simulink model "OPModel"  (R2014a)
settings: Solver=ode45  StartTime=0.0  StopTime=10  RelTol=1e-3
values from neighbouring files (symbols this model uses):
  K1 = A*x+B*r    [RongKutta.m]
  K2 = A*(x+h*K1/2)+B*r    [RongKutta.m]
undefined symbols (not defined in the file or in its folder): Kd, Ki, Kp
settings Model: Creator=李广文  LastModifiedBy=李广文

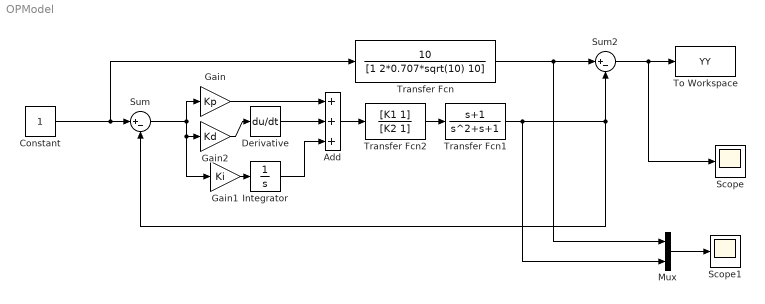
== system OPModel ==
  Add : Sum  Inputs=+++
  Constant : Constant
  Derivative : Derivative
  Gain : Gain  Gain=Kp
  Gain1 : Gain  Gain=Ki
  Gain2 : Gain  Gain=Kd
  Integrator : Integrator
  Mux : Mux  Inputs=2
  Scope : Scope
  Scope1 : Scope
      settings: YMin=0  YMax=1.5
  Sum : Sum  Inputs=|+-
  Sum2 : Sum  Inputs=|+-
  To Workspace : ToWorkspace  VariableName=YY  SampleTime=-1
  Transfer Fcn : TransferFcn  Numerator=[10]  Denominator=[1 2*0.707*sqrt(10) 10]
  Transfer Fcn1 : TransferFcn  Numerator=[1 1]  Denominator=[1 1 1]
  Transfer Fcn2 : TransferFcn  Numerator=[K1 1]  Denominator=[K2 1]
  wires:
  Constant/1 -> Transfer Fcn/1, Sum/1
  Sum/1 -> Gain/1, Gain2/1, Gain1/1
  Transfer Fcn1/1 -> Mux/2, Sum/2, Sum2/2
  Transfer Fcn/1 -> Mux/1, Sum2/1
  Sum2/1 -> Scope/1, To Workspace/1
  Mux/1 -> Scope1/1
  Gain/1 -> Add/1
  Derivative/1 -> Add/2
  Integrator/1 -> Add/3
  Gain1/1 -> Integrator/1
  Gain2/1 -> Derivative/1
  Add/1 -> Transfer Fcn2/1
  Transfer Fcn2/1 -> Transfer Fcn1/1
